simulink model "part1111"  (R2017b)
settings: Solver=VariableStepAuto  StartTime=0.0  StopTime=2  MaxStep=0.000001  RelTol=1e-3
settings Model: Creator=ras19  LastModifiedBy=drone
settings CodeAppCC: StateflowObjectComments=on

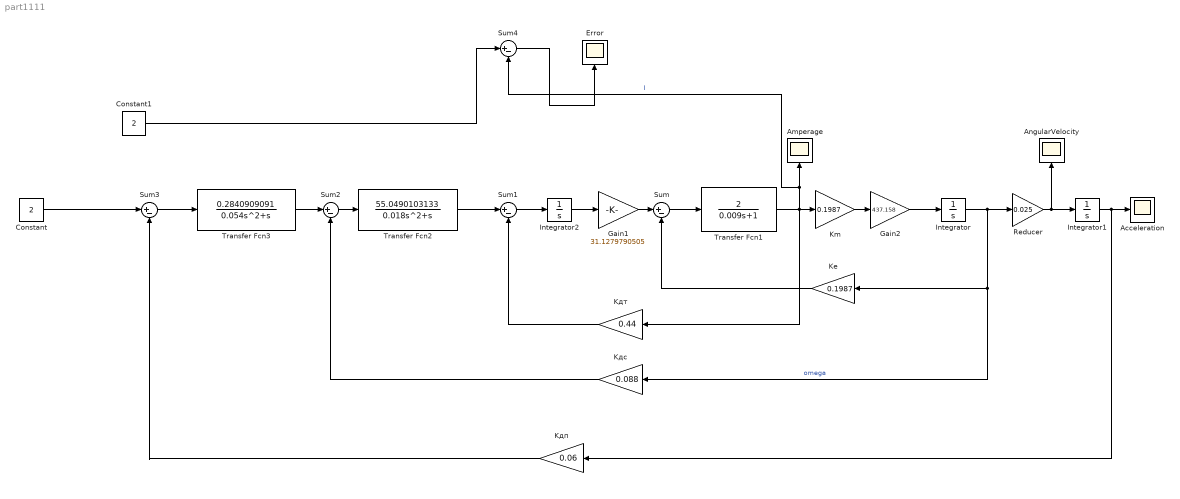
== system part1111 ==
  Acceleration : Scope
  Amperage : Scope
  AngularVelocity : Scope
  Constant : Constant  Value=2
  Constant1 : Constant  Value=2
  Error : Scope
  Gain1 : Gain  Gain=31.1279790505
  Gain2 : Gain  Gain=437.158
  Integrator : Integrator
  Integrator1 : Integrator
  Integrator2 : Integrator
  Ke : Gain  Gain=0.1987
  Km : Gain  Gain=0.1987
  Kдп : Gain  Gain=0.06
  Kдс : Gain  Gain=0.088
  Kдт : Gain  Gain=0.44
  Reducer : Gain  Gain=0.025
  Sum{,1..4} (5 alike) : Sum  Inputs=|+-
  Transfer Fcn1 : TransferFcn  Numerator=[2]  Denominator=[0.009 1]
  Transfer Fcn2 : TransferFcn  Numerator=[55.0490103133]  Denominator=[0.018 1 0]
  Transfer Fcn3 : TransferFcn  Numerator=|  Denominator=[0.054 1 0]
      | [0.2840909091
      | ]
  wires:
  Sum/1 -> Transfer Fcn1/1
  Transfer Fcn1/1 -> Kдт/1, Km/1, Sum4/2, Amperage/1  "I"
  Km/1 -> Gain2/1
  Gain2/1 -> Integrator/1
  Ke/1 -> Sum/2
  Reducer/1 -> AngularVelocity/1, Integrator1/1
  Integrator/1 -> Kдс/1, Ke/1, Reducer/1  "omega"
  Integrator1/1 -> Kдп/1, Acceleration/1
  Integrator2/1 -> Gain1/1
  Gain1/1 -> Sum/1
  Sum1/1 -> Integrator2/1
  Kдт/1 -> Sum1/2
  Sum2/1 -> Transfer Fcn2/1
  Kдс/1 -> Sum2/2
  Sum3/1 -> Transfer Fcn3/1
  Kдп/1 -> Sum3/2
  Constant/1 -> Sum3/1
  Sum4/1 -> Error/1
  Transfer Fcn2/1 -> Sum1/1
  Transfer Fcn3/1 -> Sum2/1
  Constant1/1 -> Sum4/1
